simulink model "Gecko_VR1"  (Simulink 7.6)
settings: Solver=ode3  SolverMode=SingleTasking  StartTime=0.0  StopTime=0.0008  FixedStep=1e-6  MaxStep=1e-6  MinStep=0.7e-6  RelTol=1e-3
settings Model: Creator=drofenik  LastModifiedBy=andy  BufferReuse=off
settings SolverCC: AutoInsertRateTranBlk=on  InsertRTBMode=Always
settings DataIOCC: SignalLoggingName=sigsOut
settings OptimizationCC: OptimizeBlockIOStorage=off  BufferReuse=off  ExpressionFolding=off  LocalBlockOutputs=off  InitFltsAndDblsToZero=on
settings DebuggingCC: AlgebraicLoopMsg=none  SaveWithParameterizedLinksMsg=none  SignalResolutionControl=TryResolveAllWithWarning  SolverPrmCheckMsg=none  MultiTaskDSMMsg=warning  MultiTaskCondExecSysMsg=none  StrictBusMsg=None
settings HardwareCC: TargetUnknown=on
settings RTWCC: IncludeERTFirstTime=on
settings GRTTargetCC: TargetFcnLib=ansi_tfl_tmw.mat  ModelReferenceCompliant=off  MatFileLogging=off

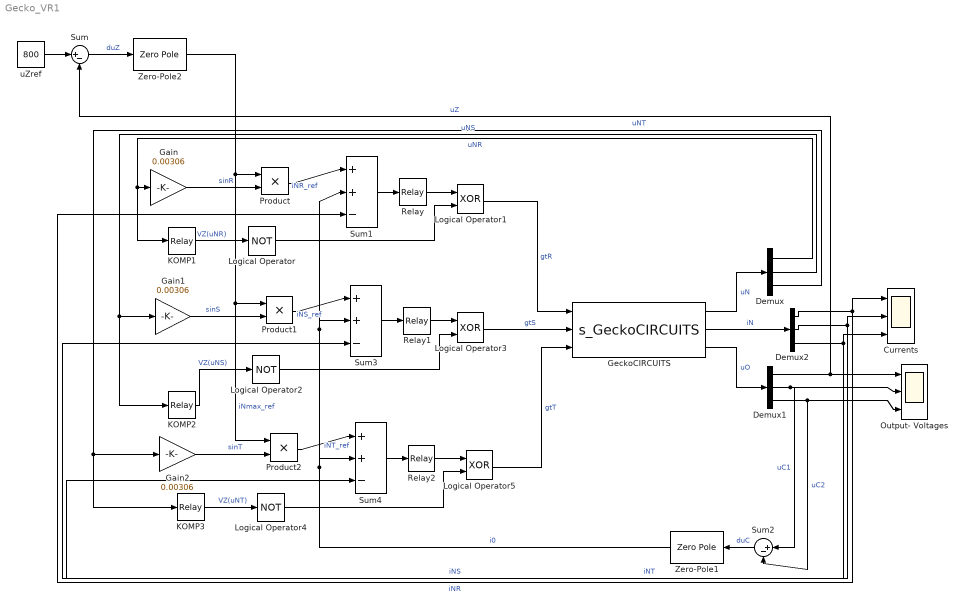
== system Gecko_VR1 ==
  Currents : Scope  NumInputPorts=3
      settings: YMin=-30~-90~-30  YMax=30~30~90
  Demux : Demux  Outputs=3
  Demux1 : Demux  Outputs=3
  Demux2 : Demux  Outputs=3
  Gain : Gain  Gain=0.00306
  Gain1 : Gain  Gain=0.00306
  Gain2 : Gain  Gain=0.00306
  GeckoCIRCUITS : S-Function  FunctionName=s_GeckoCIRCUITS  Parameters='C:/GeckoSimulink/vr1_simulink.ipes'  EnableBusSupport=off  mask{GeckoModelPath='C:/GeckoSimulink/vr1_simulink.ipes'}
      mask prompts: GeckoModelPath "Gecko-model-path (.ipes)"
      mask init:
      | inames=get_param(gcb,'InputSignalNames');
      | onames=get_param(gcb,'OutputSignalNames');
      | 
      | set_param(gcb,'Parameters', GeckoModelPath);
      | 
      | for j = 1 : length(inames)
      |     gecko.GeckoSimulink.external_setInputPortName(j-1, inames{j});
      | end
      | 
      | 
      | for j = 1 : length(onames)
      |     gecko.GeckoSimulink.external_setOutputPortName(j-1, onames{j});
      | end
      mask Display:
      | image(imread('Gecko.jpg'))
      | 
      | for j=1:length(inames)
      |     port_label('input',j,inames{j})
      | end
      | 
      | for j=1:length(onames)
      |     port_label('output',j,onames{j})
      | end
  KOMP1 : Relay  OnSwitchValue=0.001  OffSwitchValue=-0.001
  KOMP2 : Relay  OnSwitchValue=0.001  OffSwitchValue=-0.001
  KOMP3 : Relay  OnSwitchValue=0.001  OffSwitchValue=-0.001
  Logical Operator : Logic  Operator=NOT  AllPortsSameDT=off  OutDataTypeStr=boolean
  Logical Operator1 : Logic  Operator=XOR  AllPortsSameDT=off  OutDataTypeStr=boolean
  Logical Operator2 : Logic  Operator=NOT  AllPortsSameDT=off  OutDataTypeStr=boolean
  Logical Operator3 : Logic  Operator=XOR  AllPortsSameDT=off  OutDataTypeStr=boolean
  Logical Operator4 : Logic  Operator=NOT  AllPortsSameDT=off  OutDataTypeStr=boolean
  Logical Operator5 : Logic  Operator=XOR  AllPortsSameDT=off  OutDataTypeStr=boolean
  Output- Voltages : Scope  NumInputPorts=3
      settings: YMin=535~252.5~282.5  YMax=577.5~275~305
  Product : Product  RndMeth=Zero
  Product1 : Product  RndMeth=Zero
  Product2 : Product  RndMeth=Zero
  Relay : Relay  OnSwitchValue=1.5  OffSwitchValue=-1.5
  Relay1 : Relay  OnSwitchValue=1.5  OffSwitchValue=-1.5
  Relay2 : Relay  OnSwitchValue=1.5  OffSwitchValue=-1.5
  Sum : Sum  Inputs=|+-
  Sum1 : Sum  Inputs=|++-
  Sum2 : Sum  Inputs=|+-
  Sum3 : Sum  Inputs=|++-
  Sum4 : Sum  Inputs=|++-
  Zero-Pole1 : ZeroPole  Zeros=[-50]  Poles=[0]  Gain=[2]
  Zero-Pole2 : ZeroPole  Zeros=[-50]  Poles=[0]  Gain=[2]
  uZref : Constant  Value=800
  wires:
  uZref/1 -> Sum/1
  Sum/1 -> Zero-Pole2/1  "duZ"
  Zero-Pole2/1 -> Product/1, Product1/1, Product2/1  "iNmax_ref"
  KOMP1/1 -> Logical Operator/1  "VZ(uNR)"
  Gain/1 -> Product/2  "sinR"
  Product/1 -> Sum1/1  "iNR_ref"
  Sum1/1 -> Relay/1
  Relay/1 -> Logical Operator1/1
  Logical Operator/1 -> Logical Operator1/2
  KOMP2/1 -> Logical Operator2/1  "VZ(uNS)"
  Gain1/1 -> Product1/2  "sinS"
  Product1/1 -> Sum3/1  "iNS_ref"
  Sum3/1 -> Relay1/1
  Relay1/1 -> Logical Operator3/1
  Logical Operator2/1 -> Logical Operator3/2
  KOMP3/1 -> Logical Operator4/1  "VZ(uNT)"
  Gain2/1 -> Product2/2  "sinT"
  Product2/1 -> Sum4/1  "iNT_ref"
  Sum4/1 -> Relay2/1
  Relay2/1 -> Logical Operator5/1
  Logical Operator4/1 -> Logical Operator5/2
  Demux2/1 -> Sum1/3, Currents/1  "iNR"
  Demux2/2 -> Sum3/3, Currents/2  "iNS"
  Demux2/3 -> Sum4/3, Currents/3  "iNT"
  Demux1/1 -> Sum/2, Output- Voltages/1  "uZ"
  Demux1/2 -> Sum2/1, Output- Voltages/2  "uC1"
  Demux1/3 -> Sum2/2, Output- Voltages/3  "uC2"
  Zero-Pole1/1 -> Sum1/2, Sum3/2, Sum4/2  "i0"
  Sum2/1 -> Zero-Pole1/1  "duC"
  Demux/1 -> Gain/1, KOMP1/1  "uNR"
  Demux/2 -> KOMP2/1, Gain1/1  "uNS"
  Demux/3 -> Gain2/1, KOMP3/1  "uNT"
  Logical Operator1/1 -> GeckoCIRCUITS/1  "gtR"
  Logical Operator5/1 -> GeckoCIRCUITS/3  "gtT"
  Logical Operator3/1 -> GeckoCIRCUITS/2  "gtS"
  GeckoCIRCUITS/1 -> Demux/1  "uN"
  GeckoCIRCUITS/3 -> Demux1/1  "uO"
  GeckoCIRCUITS/2 -> Demux2/1  "iN"
